simulink model "modelLab3"  (R2022b)
settings: Solver=VariableStepAuto  StartTime=0.0  StopTime=60  RelTol=1e-3
values from neighbouring files (symbols this model uses):
  A = [0, 0, 1, 0 ... (first row only)    [initLab3.m]
  B = [0, 0 ... (first row only)    [initLab3.m]
  C = eye(4)    [initLab3.m]
  cmdPitchFrq = 1 ./ 20    [initLab3.m]
  cmdPitchMag = 0.34    [initLab3.m]
  cmdYawRate = 1.2566    [initLab3.m]
  D = zeros(4,2)    [initLab3.m]
  den = den{1}    [initLab3.m]
  K = place(phi, gamma, zpoles)    [initLab3.m]
  num = num{1}    [initLab3.m]
  r2d = 180 ./ pi    [initLab3.m]
  T = min(Ts ./ (20 .* n), pi ./ (5 .* 1.2982))    [initLab3.m]
  x0 = [0; 0; 0; 0]    [initLab3.m]
libraries: simulink x1
settings Model: Creator=fwah  LastModifiedBy=fwah

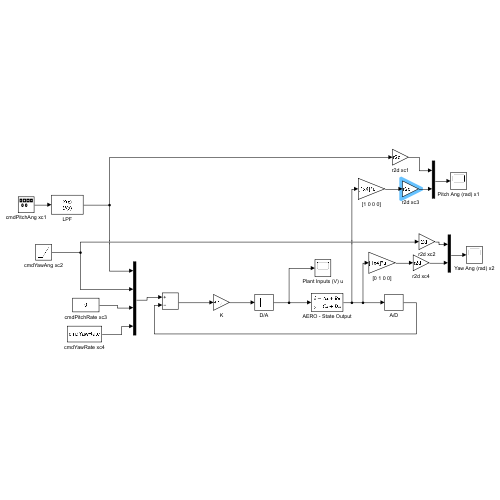
[thumbnail: Simulink's stored preview of the top-level diagram]
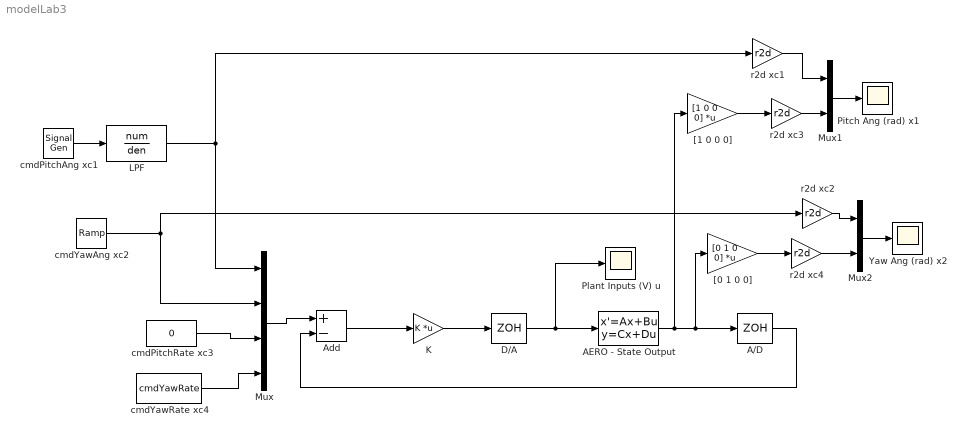
== system modelLab3 ==
  A/D : ZeroOrderHold  SampleTime=T
  AERO - State Output : StateSpace  A=A  B=B  C=C  D=D  InitialCondition=x0
  Add : Sum  Inputs=+-
  D/A : ZeroOrderHold  SampleTime=T
  K : Gain  Gain=K  Multiplication=Matrix(K*u)
  LPF : DiscreteTransferFcn  Numerator=num  Denominator=den  SampleTime=T
  Mux : Mux
  Mux1 : Mux  Inputs=2
  Mux2 : Mux  Inputs=2
  Pitch Ang (rad) x1 : Scope
  Plant Inputs (V) u : Scope
  Yaw Ang (rad) x2 : Scope
  "[0 1 0 0]" : Gain  Gain=[0 1 0 0]  Multiplication=Matrix(K*u)
  "[1 0 0 0]" : Gain  Gain=[1 0 0 0]  Multiplication=Matrix(K*u)
  cmdPitchAng xc1 : SignalGenerator  WaveForm=square  Amplitude=cmdPitchMag  Frequency=cmdPitchFrq
  cmdPitchRate xc3 : Constant  Value=0
  cmdYawAng xc2 : simulink/Sources/Ramp  slope=cmdYawRate  start=0  InitialOutput=0
  cmdYawRate xc4 : Constant  Value=cmdYawRate
  r2d xc{1..4} (4 alike) : Gain  Gain=r2d
  wires:
  cmdYawRate xc4/1 -> Mux/4
  K/1 -> D/A/1
  Mux/1 -> Add/1
  cmdPitchAng xc1/1 -> LPF/1
  Add/1 -> K/1
  D/A/1 -> AERO - State Output/1, Plant Inputs (V) u/1
  cmdYawAng xc2/1 -> Mux/2, r2d xc2/1
  cmdPitchRate xc3/1 -> Mux/3
  LPF/1 -> Mux/1, r2d xc1/1
  AERO - State Output/1 -> A/D/1, "[0 1 0 0]"/1, "[1 0 0 0]"/1
  A/D/1 -> Add/2
  r2d xc1/1 -> Mux1/1
  r2d xc2/1 -> Mux2/1
  Mux1/1 -> Pitch Ang (rad) x1/1
  Mux2/1 -> Yaw Ang (rad) x2/1
  "[0 1 0 0]"/1 -> r2d xc4/1
  r2d xc4/1 -> Mux2/2
  "[1 0 0 0]"/1 -> r2d xc3/1
  r2d xc3/1 -> Mux1/2
